simulink model "simulinkmodel"  (R2023a)
settings: Solver=ode4  StartTime=0.0  StopTime=250.0  FixedStep=1e-3  RelTol=1e-3
values from neighbouring files (symbols this model uses):
  ARw = 7.9456    [EOMs_of_AC.m]    (also in constants_simulinkmodel.m)
  b = 9.16    [EOMs_of_AC.m]    (also in constants_simulinkmodel.m)
  c = 1.3333    [EOMs_of_AC.m]    (also in constants_simulinkmodel.m)
  CDf = .005    (= 0.005)    [EOMs_of_AC.m]    (also in constants_simulinkmodel.m)
  CDmint = .002    (= 0.002)    [EOMs_of_AC.m]    (also in constants_simulinkmodel.m)
  CDminvt = .001    (= 0.001)    [EOMs_of_AC.m]    (also in constants_simulinkmodel.m)
  CDminw = .011    (= 0.011)    [EOMs_of_AC.m]    (also in constants_simulinkmodel.m)
  cgt = 3.5    [EOMs_of_AC.m]    (also in constants_simulinkmodel.m)
  cgvt = cgt    (= 3.5)    [EOMs_of_AC.m]    (also in constants_simulinkmodel.m)
  cgw = -.416    (= -0.416)    [EOMs_of_AC.m]    (also in constants_simulinkmodel.m)
  CLat = .76    (= 0.76)    [EOMs_of_AC.m]    (also in constants_simulinkmodel.m)
  CLavt = .0969    (= 0.0969)    [EOMs_of_AC.m]    (also in constants_simulinkmodel.m)
  CLaw = 4.59    [EOMs_of_AC.m]    (also in constants_simulinkmodel.m)
  Clb = -.1    (= -0.1)    [EOMs_of_AC.m]    (also in constants_simulinkmodel.m)
  Clda = 0.244    [EOMs_of_AC.m]    (also in constants_simulinkmodel.m)
  CLow = .421    (= 0.421)    [EOMs_of_AC.m]    (also in constants_simulinkmodel.m)
  Clr = .01    (= 0.01)    [EOMs_of_AC.m]    (also in constants_simulinkmodel.m)
  Cmaf = .114    (= 0.114)    [EOMs_of_AC.m]    (also in constants_simulinkmodel.m)
  Cmw = -0.005    [EOMs_of_AC.m]    (also in constants_simulinkmodel.m)
  Cnda = -0.0128    [EOMs_of_AC.m]    (also in constants_simulinkmodel.m)
  e = .75    (= 0.75)    [EOMs_of_AC.m]    (also in constants_simulinkmodel.m)
  g = 32.17    [EOMs_of_AC.m]    (also in constants_simulinkmodel.m)
  it = 2*d2r    (= 0.0349065850399)    [EOMs_of_AC.m]    (also in constants_simulinkmodel.m = 0.034906585)
  Ixx = 1.9480    (= 1.948)    [EOMs_of_AC.m]    (also in constants_simulinkmodel.m)
  Iyy = 1.5523    [EOMs_of_AC.m]    (also in constants_simulinkmodel.m)
  Izz = 1.9166    [EOMs_of_AC.m]    (also in constants_simulinkmodel.m)
  Kt = .446    (= 0.446)    [EOMs_of_AC.m]    (also in constants_simulinkmodel.m)
  lambda = .72955    (= 0.72955)    [EOMs_of_AC.m]    (also in constants_simulinkmodel.m)
  m = .487669    (= 0.487669)    [EOMs_of_AC.m]    (also in constants_simulinkmodel.m)
  nt = 1    [EOMs_of_AC.m]    (also in constants_simulinkmodel.m)
  nvt = nt    (= 1)    [EOMs_of_AC.m]    (also in constants_simulinkmodel.m)
  rho = .0023081    (= 0.0023081)    [EOMs_of_AC.m]    (also in constants_simulinkmodel.m)
  S = 10.56    [EOMs_of_AC.m]    (also in constants_simulinkmodel.m)
  St = S    (= 10.56)    [EOMs_of_AC.m]    (also in constants_simulinkmodel.m)
  Svt = S    (= 10.56)    [EOMs_of_AC.m]    (also in constants_simulinkmodel.m)
  Te = .422    (= 0.422)    [EOMs_of_AC.m]    (also in constants_simulinkmodel.m)
  Tr = .434    (= 0.434)    [EOMs_of_AC.m]    (also in constants_simulinkmodel.m)
undefined symbols (not defined in the file or in its folder): JSBSim, Rascal110, x_initial
libraries: simulink_extras x12, aerolibfltsims x2, aerolibanimutils x1
(part 2 of 2)

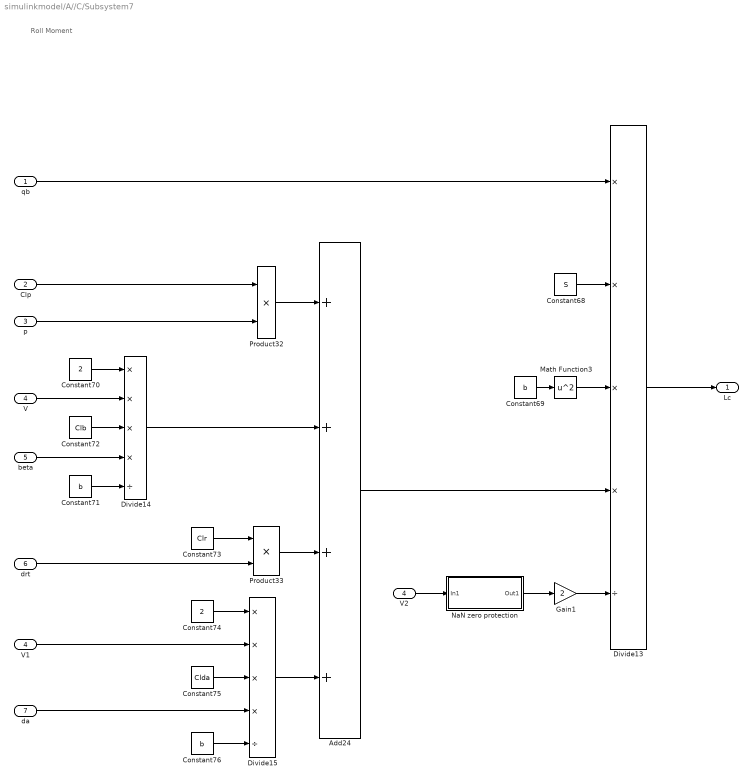
== system simulinkmodel/A//C/Subsystem7 ==
  note: Roll Moment
  qb : Inport
  Clp : Inport  Port=2
  p : Inport  Port=3
  V : Inport  Port=4
  beta : Inport  Port=5
  drt : Inport  Port=6
  da : Inport  Port=7
  Add24 : Sum  Inputs=++++
  Constant68 : Constant  Value=S
  Constant69 : Constant  Value=b
  Constant70 : Constant  Value=2
  Constant71 : Constant  Value=b
  Constant72 : Constant  Value=Clb
  Constant73 : Constant  Value=Clr
  Constant74 : Constant  Value=2
  Constant75 : Constant  Value=Clda
  Constant76 : Constant  Value=b
  Divide13 : Product  Inputs=****/
  Divide14 : Product  Inputs=****/
  Divide15 : Product  Inputs=****/
  Gain1 : Gain  Gain=2
  Math Function3 : Math  Operator=square
  NaN zero protection : Subsystem
  Product32 : Product
  Product33 : Product
  V1 : InportShadow  Port=4
  V2 : InportShadow  Port=4
  Lc : Outport
  wires:
  Add24/1 -> Divide13/4
  Constant72/1 -> Divide14/3
  Math Function3/1 -> Divide13/3
  Constant68/1 -> Divide13/2
  Gain1/1 -> Divide13/5
  Constant73/1 -> Product33/1
  Constant75/1 -> Divide15/3
  Divide14/1 -> Add24/2
  Constant74/1 -> Divide15/1
  Constant69/1 -> Math Function3/1
  Constant76/1 -> Divide15/5
  Product33/1 -> Add24/3
  Divide15/1 -> Add24/4
  qb/1 -> Divide13/1
  Constant71/1 -> Divide14/5
  Product32/1 -> Add24/1
  NaN zero protection/1(Out1) -> Gain1/1
  Constant70/1 -> Divide14/1
  Divide13/1 -> Lc/1
  drt/1 -> Product33/2
  beta/1 -> Divide14/4
  V/1 -> Divide14/2
  da/1 -> Divide15/4
  V1/1 -> Divide15/2
  Clp/1 -> Product32/1
  V2/1 -> NaN zero protection/1(In1)
  p/1 -> Product32/2

== system simulinkmodel/A//C/Subsystem8 ==
  note: Acceleration
  D : Inport
  beta : Inport  Port=2
  Y : Inport  Port=3
  T : Inport  Port=4
  alpha : Inport  Port=5
  gamma : Inport  Port=6
  Add25 : Sum  Inputs=+-
  Add26 : Sum  Inputs=-++
  Constant77 : Constant  Value=g
  Constant78 : Constant  Value=m
  Divide16 : Product  Inputs=*/
  Product34 : Product
  Product35 : Product
  Product36 : Product
  Product37 : Product  Inputs=3
  Trigonometric Function10 : Trigonometry
  Trigonometric Function11 : Trigonometry  Operator=cos
  Trigonometric Function12 : Trigonometry  Operator=cos
  Trigonometric Function8 : Trigonometry
  Trigonometric Function9 : Trigonometry  Operator=cos
  beta1 : InportShadow  Port=2
  beta2 : InportShadow  Port=2
  V_dot : Outport
  wires:
  Trigonometric Function8/1 -> Product34/2
  Constant77/1 -> Product34/1
  Product34/1 -> Add25/2
  Trigonometric Function12/1 -> Product37/3
  Product36/1 -> Add26/2
  Constant78/1 -> Divide16/2
  Divide16/1 -> Add25/1
  Product35/1 -> Add26/1
  Trigonometric Function11/1 -> Product37/2
  Product37/1 -> Add26/3
  Add26/1 -> Divide16/1
  Y/1 -> Product36/1
  Trigonometric Function10/1 -> Product36/2
  Trigonometric Function9/1 -> Product35/2
  Add25/1 -> V_dot/1
  D/1 -> Product35/1
  beta1/1 -> Trigonometric Function10/1
  gamma/1 -> Trigonometric Function8/1
  T/1 -> Product37/1
  beta/1 -> Trigonometric Function9/1
  beta2/1 -> Trigonometric Function11/1
  alpha/1 -> Trigonometric Function12/1

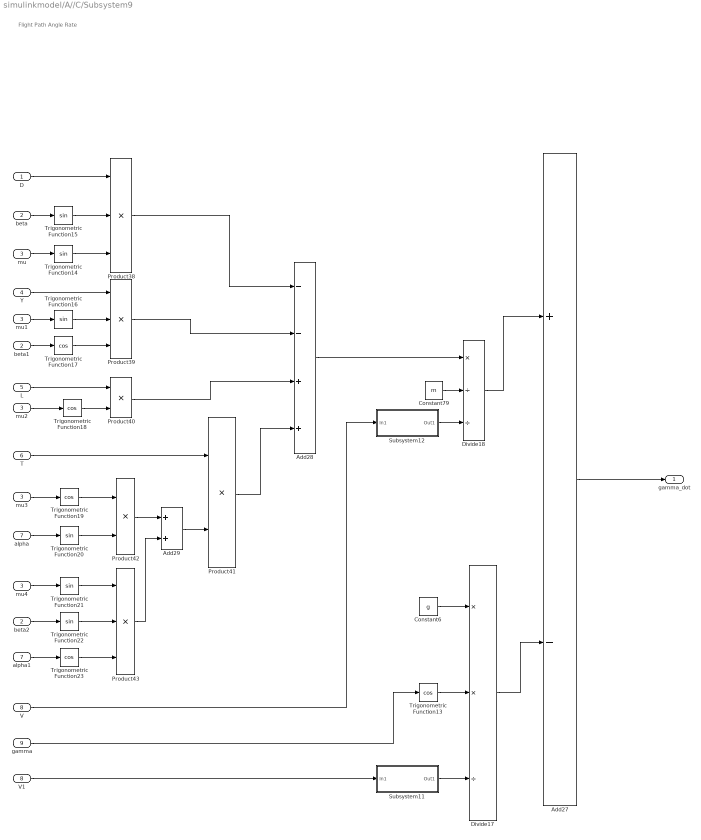
== system simulinkmodel/A//C/Subsystem9 ==
  note: Flight Path Angle Rate
  D : Inport
  beta : Inport  Port=2
  mu : Inport  Port=3
  Y : Inport  Port=4
  L : Inport  Port=5
  T : Inport  Port=6
  alpha : Inport  Port=7
  V : Inport  Port=8
  gamma : Inport  Port=9
  Add27 : Sum  Inputs=+-
  Add28 : Sum  Inputs=--++
  Add29 : Sum
  Constant6 : Constant  Value=g
  Constant79 : Constant  Value=m
  Divide17 : Product  Inputs=**/
  Divide18 : Product  Inputs=*//
  Product38 : Product  Inputs=3
  Product39 : Product  Inputs=3
  Product40 : Product
  Product41 : Product
  Product42 : Product
  Product43 : Product  Inputs=3
  Subsystem11 : Subsystem
  Subsystem12 : Subsystem
  Trigonometric Function{13,17..19,23} (5 alike) : Trigonometry  Operator=cos
  Trigonometric Function{14..16,20..22} (6 alike) : Trigonometry
  V1 : InportShadow  Port=8
  alpha1 : InportShadow  Port=7
  beta1 : InportShadow  Port=2
  beta2 : InportShadow  Port=2
  mu{1..4} (4 alike) : InportShadow  Port=3
  gamma_dot : Outport
  wires:
  alpha/1 -> Trigonometric Function20/1
  Product41/1 -> Add28/4
  Product38/1 -> Add28/1
  Constant6/1 -> Divide17/1
  Divide17/1 -> Add27/2
  mu2/1 -> Trigonometric Function18/1
  Trigonometric Function23/1 -> Product43/3
  Add29/1 -> Product41/2
  Trigonometric Function15/1 -> Product38/2
  Trigonometric Function14/1 -> Product38/3
  Trigonometric Function18/1 -> Product40/2
  Product39/1 -> Add28/2
  mu1/1 -> Trigonometric Function16/1
  Product40/1 -> Add28/3
  Trigonometric Function16/1 -> Product39/2
  V1/1 -> Subsystem11/1(In1)
  alpha1/1 -> Trigonometric Function23/1
  Add28/1 -> Divide18/1
  mu/1 -> Trigonometric Function14/1
  Trigonometric Function17/1 -> Product39/3
  Constant79/1 -> Divide18/2
  Subsystem11/1(Out1) -> Divide17/3
  Trigonometric Function22/1 -> Product43/2
  beta2/1 -> Trigonometric Function22/1
  Product43/1 -> Add29/2
  L/1 -> Product40/1
  Product42/1 -> Add29/1
  Divide18/1 -> Add27/1
  Trigonometric Function20/1 -> Product42/2
  Trigonometric Function13/1 -> Divide17/2
  Trigonometric Function21/1 -> Product43/1
  Trigonometric Function19/1 -> Product42/1
  mu3/1 -> Trigonometric Function19/1
  Subsystem12/1(Out1) -> Divide18/3
  gamma/1 -> Trigonometric Function13/1
  beta/1 -> Trigonometric Function15/1
  D/1 -> Product38/1
  T/1 -> Product41/1
  beta1/1 -> Trigonometric Function17/1
  V/1 -> Subsystem12/1(In1)
  mu4/1 -> Trigonometric Function21/1
  Add27/1 -> gamma_dot/1
  Y/1 -> Product39/1

== system simulinkmodel/Subsystem1/Subsystem ==
  note: Meridian Radius
  latitude : Inport
  Add : Sum  Inputs=+-
  Add1 : Sum  Inputs=+-
  Constant : Constant
  Constant1 : Constant
  Constant2 : Constant  Value=3/2
  Divide : Product  Inputs=**/
  Math Function : Math  Operator=square
  Math Function1 : Math  Operator=square
  Math Function2 : Math  Operator=square
  Math Function3 : Math  Operator=pow
  Product : Product
  Trigonometric Function : Trigonometry
  a (equitorial radius) : Constant  Value=6378137
  e (first eccentricity) : Constant  Value=0.081819190842622
  e (first eccentricity)1 : Constant  Value=0.081819190842622
  M : Outport
  wires:
  Constant1/1 -> Add1/1
  Add/1 -> Divide/2
  Add1/1 -> Math Function3/1
  Constant2/1 -> Math Function3/2
  Product/1 -> Add1/2
  a (equitorial radius)/1 -> Divide/1
  e (first eccentricity)1/1 -> Math Function1/1
  latitude/1 -> Trigonometric Function/1
  Math Function/1 -> Add/2
  Constant/1 -> Add/1
  Trigonometric Function/1 -> Math Function2/1
  e (first eccentricity)/1 -> Math Function/1
  Math Function1/1 -> Product/1
  Math Function2/1 -> Product/2
  Math Function3/1 -> Divide/3
  Divide/1 -> M/1

== system simulinkmodel/Subsystem1/Subsystem1 ==
  note: Prime Vertical Radius
  latitude : Inport
  Add1 : Sum  Inputs=+-
  Constant1 : Constant
  Constant2 : Constant  Value=1/2
  Divide : Product  Inputs=*/
  Math Function1 : Math  Operator=square
  Math Function2 : Math  Operator=square
  Math Function3 : Math  Operator=pow
  Product : Product
  Trigonometric Function : Trigonometry
  a (equitorial radius) : Constant  Value=6378137
  e (first eccentricity) : Constant  Value=0.081819190842622
  N : Outport
  wires:
  Math Function1/1 -> Product/1
  Product/1 -> Add1/2
  Constant2/1 -> Math Function3/2
  Constant1/1 -> Add1/1
  Add1/1 -> Math Function3/1
  latitude/1 -> Trigonometric Function/1
  Math Function3/1 -> Divide/2
  Math Function2/1 -> Product/2
  Trigonometric Function/1 -> Math Function2/1
  e (first eccentricity)/1 -> Math Function1/1
  a (equitorial radius)/1 -> Divide/1
  Divide/1 -> N/1

== system simulinkmodel/Subsystem1/Subsystem2 ==
  note: Latitude Rate
  n_dot : Inport
  M : Inport  Port=2
  h : Inport  Port=3
  Add : Sum
  Divide : Product  Inputs=*/
  ft2m1 : Gain  Gain=0.3048
  latitude_dot : Outport
  wires:
  Add/1 -> Divide/2
  n_dot/1 -> ft2m1/1
  Divide/1 -> latitude_dot/1
  M/1 -> Add/1
  ft2m1/1 -> Divide/1
  h/1 -> Add/2

== system simulinkmodel/Subsystem1/Subsystem3 ==
  note: Longitude Rate
  e_dot : Inport
  N : Inport  Port=2
  h : Inport  Port=3
  latitude : Inport  Port=4
  Add : Sum
  Divide : Product  Inputs=*//
  Gain1 : Gain  Gain=0.3048
  Trigonometric Function : Trigonometry  Operator=cos
  longitude_dot : Outport
  wires:
  Trigonometric Function/1 -> Divide/3
  Divide/1 -> longitude_dot/1
  Add/1 -> Divide/2
  e_dot/1 -> Gain1/1
  latitude/1 -> Trigonometric Function/1
  N/1 -> Add/1
  Gain1/1 -> Divide/1
  h/1 -> Add/2

== system simulinkmodel/Subsystem1/Subsystem4 ==
  note: Altitude Rate
  d_dot : Inport
  Gain : Gain  Gain=-1
  ft2m : Gain  Gain=0.3048
  h_dot : Outport
  wires:
  d_dot/1 -> ft2m/1
  Gain/1 -> h_dot/1
  ft2m/1 -> Gain/1

== system simulinkmodel/A//C/Subsystem10/Subsystem13 ==
  In1 : Inport
  Constant : Constant  Value=1e-8
  Relational Operator : RelationalOperator  Operator=>  OutDataTypeStr=boolean  RndMeth=Simplest  InputSameDT=off
  Switch : Switch  Criteria=u2 ~= 0  SaturateOnIntegerOverflow=off  InputSameDT=off
  Out1 : Outport
  wires:
  Switch/1 -> Out1/1
  Relational Operator/1 -> Switch/2
  Constant/1 -> Relational Operator/2, Switch/3
  In1/1 -> Relational Operator/1, Switch/1

== system simulinkmodel/A//C/Subsystem10/Subsystem14 ==
  In1 : Inport
  Constant : Constant  Value=1e-8
  Relational Operator : RelationalOperator  Operator=>  OutDataTypeStr=boolean  RndMeth=Simplest  InputSameDT=off
  Switch : Switch  Criteria=u2 ~= 0  SaturateOnIntegerOverflow=off  InputSameDT=off
  Out1 : Outport
  wires:
  In1/1 -> Switch/1, Relational Operator/1
  Constant/1 -> Switch/3, Relational Operator/2
  Relational Operator/1 -> Switch/2
  Switch/1 -> Out1/1

== system simulinkmodel/A//C/Subsystem14/Subsystem15 ==
  In1 : Inport
  Constant : Constant  Value=1e-8
  Relational Operator : RelationalOperator  Operator=>  OutDataTypeStr=boolean  RndMeth=Simplest  InputSameDT=off
  Switch : Switch  Criteria=u2 ~= 0  SaturateOnIntegerOverflow=off  InputSameDT=off
  Out1 : Outport
  wires:
  Switch/1 -> Out1/1
  Relational Operator/1 -> Switch/2
  Constant/1 -> Relational Operator/2, Switch/3
  In1/1 -> Relational Operator/1, Switch/1

== system simulinkmodel/A//C/Subsystem14/Subsystem16 ==
  In1 : Inport
  Constant : Constant  Value=1e-8
  Relational Operator : RelationalOperator  Operator=>  OutDataTypeStr=boolean  RndMeth=Simplest  InputSameDT=off
  Switch : Switch  Criteria=u2 ~= 0  SaturateOnIntegerOverflow=off  InputSameDT=off
  Out1 : Outport
  wires:
  In1/1 -> Switch/1, Relational Operator/1
  Constant/1 -> Switch/3, Relational Operator/2
  Relational Operator/1 -> Switch/2
  Switch/1 -> Out1/1

== system simulinkmodel/A//C/Subsystem15/Subsystem17 ==
  In1 : Inport
  Constant : Constant  Value=1e-8
  Relational Operator : RelationalOperator  Operator=>  OutDataTypeStr=boolean  RndMeth=Simplest  InputSameDT=off
  Switch : Switch  Criteria=u2 ~= 0  SaturateOnIntegerOverflow=off  InputSameDT=off
  Out1 : Outport
  wires:
  In1/1 -> Switch/1, Relational Operator/1
  Constant/1 -> Switch/3, Relational Operator/2
  Relational Operator/1 -> Switch/2
  Switch/1 -> Out1/1

== system simulinkmodel/A//C/Subsystem15/Subsystem18 ==
  V : Inport
  Constant : Constant  Value=1e-8
  Relational Operator : RelationalOperator  Operator=>  OutDataTypeStr=boolean  RndMeth=Simplest  InputSameDT=off
  Switch : Switch  Criteria=u2 ~= 0  SaturateOnIntegerOverflow=off  InputSameDT=off
  Out1 : Outport
  wires:
  Switch/1 -> Out1/1
  Relational Operator/1 -> Switch/2
  Constant/1 -> Relational Operator/2, Switch/3
  V/1 -> Relational Operator/1, Switch/1

== system simulinkmodel/A//C/Subsystem2/Subsystem1 ==
  In1 : Inport
  Constant : Constant  Value=1e-8
  Relational Operator : RelationalOperator  Operator=>  OutDataTypeStr=boolean  RndMeth=Simplest  InputSameDT=off
  Switch : Switch  Criteria=u2 ~= 0  SaturateOnIntegerOverflow=off  InputSameDT=off
  Out1 : Outport
  wires:
  Switch/1 -> Out1/1
  Relational Operator/1 -> Switch/2
  Constant/1 -> Relational Operator/2, Switch/3
  In1/1 -> Relational Operator/1, Switch/1

== system simulinkmodel/A//C/Subsystem25/Subsystem2 ==
  In1 : Inport
  Constant : Constant  Value=1e-8
  Relational Operator : RelationalOperator  Operator=>  OutDataTypeStr=boolean  RndMeth=Simplest  InputSameDT=off
  Switch : Switch  Criteria=u2 ~= 0  SaturateOnIntegerOverflow=off  InputSameDT=off
  Out1 : Outport
  wires:
  In1/1 -> Switch/1, Relational Operator/1
  Constant/1 -> Switch/3, Relational Operator/2
  Relational Operator/1 -> Switch/2
  Switch/1 -> Out1/1

== system simulinkmodel/A//C/Subsystem3/Subsystem5 ==
  In1 : Inport
  Constant : Constant  Value=1e-8
  Relational Operator : RelationalOperator  Operator=>  OutDataTypeStr=boolean  RndMeth=Simplest  InputSameDT=off
  Switch : Switch  Criteria=u2 ~= 0  SaturateOnIntegerOverflow=off  InputSameDT=off
  Out1 : Outport
  wires:
  In1/1 -> Switch/1, Relational Operator/1
  Constant/1 -> Switch/3, Relational Operator/2
  Relational Operator/1 -> Switch/2
  Switch/1 -> Out1/1

== system simulinkmodel/A//C/Subsystem3/Subsystem6 ==
  In1 : Inport
  Constant : Constant  Value=1e-8
  Relational Operator : RelationalOperator  Operator=>  OutDataTypeStr=boolean  RndMeth=Simplest  InputSameDT=off
  Switch : Switch  Criteria=u2 ~= 0  SaturateOnIntegerOverflow=off  InputSameDT=off
  Out1 : Outport
  wires:
  Switch/1 -> Out1/1
  Relational Operator/1 -> Switch/2
  Constant/1 -> Relational Operator/2, Switch/3
  In1/1 -> Relational Operator/1, Switch/1

== system simulinkmodel/A//C/Subsystem35/Subsystem3 ==
  In1 : Inport
  Constant : Constant  Value=1e-8
  Relational Operator : RelationalOperator  Operator=>  OutDataTypeStr=boolean  RndMeth=Simplest  InputSameDT=off
  Switch : Switch  Criteria=u2 ~= 0  SaturateOnIntegerOverflow=off  InputSameDT=off
  Out1 : Outport
  wires:
  Switch/1 -> Out1/1
  Relational Operator/1 -> Switch/2
  Constant/1 -> Relational Operator/2, Switch/3
  In1/1 -> Relational Operator/1, Switch/1

== system simulinkmodel/A//C/Subsystem35/Subsystem4 ==
  In1 : Inport
  Constant : Constant  Value=1e-8
  Relational Operator : RelationalOperator  Operator=>  OutDataTypeStr=boolean  RndMeth=Simplest  InputSameDT=off
  Switch : Switch  Criteria=u2 ~= 0  SaturateOnIntegerOverflow=off  InputSameDT=off
  Out1 : Outport
  wires:
  In1/1 -> Switch/1, Relational Operator/1
  Constant/1 -> Switch/3, Relational Operator/2
  Relational Operator/1 -> Switch/2
  Switch/1 -> Out1/1

== system simulinkmodel/A//C/Subsystem36/Subsystem19 ==
  In1 : Inport
  Constant : Constant  Value=1e-8
  Relational Operator : RelationalOperator  Operator=>  OutDataTypeStr=boolean  RndMeth=Simplest  InputSameDT=off
  Switch : Switch  Criteria=u2 ~= 0  SaturateOnIntegerOverflow=off  InputSameDT=off
  Out1 : Outport
  wires:
  Switch/1 -> Out1/1
  Relational Operator/1 -> Switch/2
  Constant/1 -> Relational Operator/2, Switch/3
  In1/1 -> Relational Operator/1, Switch/1

== system simulinkmodel/A//C/Subsystem4/Subsystem7 ==
  In1 : Inport
  Constant : Constant  Value=1e-8
  Relational Operator : RelationalOperator  Operator=>  OutDataTypeStr=boolean  RndMeth=Simplest  InputSameDT=off
  Switch : Switch  Criteria=u2 ~= 0  SaturateOnIntegerOverflow=off  InputSameDT=off
  Out1 : Outport
  wires:
  In1/1 -> Switch/1, Relational Operator/1
  Constant/1 -> Switch/3, Relational Operator/2
  Relational Operator/1 -> Switch/2
  Switch/1 -> Out1/1

== system simulinkmodel/A//C/Subsystem5/Subsystem8 ==
  In1 : Inport
  Constant : Constant  Value=1e-8
  Relational Operator : RelationalOperator  Operator=>  OutDataTypeStr=boolean  RndMeth=Simplest  InputSameDT=off
  Switch : Switch  Criteria=u2 ~= 0  SaturateOnIntegerOverflow=off  InputSameDT=off
  Out1 : Outport
  wires:
  In1/1 -> Switch/1, Relational Operator/1
  Constant/1 -> Switch/3, Relational Operator/2
  Relational Operator/1 -> Switch/2
  Switch/1 -> Out1/1

== system simulinkmodel/A//C/Subsystem5/Subsystem9 ==
  In1 : Inport
  Constant : Constant  Value=1e-8
  Relational Operator : RelationalOperator  Operator=>  OutDataTypeStr=boolean  RndMeth=Simplest  InputSameDT=off
  Switch : Switch  Criteria=u2 ~= 0  SaturateOnIntegerOverflow=off  InputSameDT=off
  Out1 : Outport
  wires:
  Switch/1 -> Out1/1
  Relational Operator/1 -> Switch/2
  Constant/1 -> Relational Operator/2, Switch/3
  In1/1 -> Relational Operator/1, Switch/1

== system simulinkmodel/A//C/Subsystem6/Subsystem10 ==
  In1 : Inport
  Constant : Constant  Value=1e-8
  Relational Operator : RelationalOperator  Operator=>  OutDataTypeStr=boolean  RndMeth=Simplest  InputSameDT=off
  Switch : Switch  Criteria=u2 ~= 0  SaturateOnIntegerOverflow=off  InputSameDT=off
  Out1 : Outport
  wires:
  In1/1 -> Switch/1, Relational Operator/1
  Constant/1 -> Switch/3, Relational Operator/2
  Relational Operator/1 -> Switch/2
  Switch/1 -> Out1/1

== system simulinkmodel/A//C/Subsystem7/NaN zero protection ==
  In1 : Inport
  Constant : Constant  Value=1e-8
  Relational Operator : RelationalOperator  Operator=>  OutDataTypeStr=boolean  RndMeth=Simplest  InputSameDT=off
  Switch : Switch  Criteria=u2 ~= 0  SaturateOnIntegerOverflow=off  InputSameDT=off
  Out1 : Outport
  wires:
  Switch/1 -> Out1/1
  Relational Operator/1 -> Switch/2
  Constant/1 -> Relational Operator/2, Switch/3
  In1/1 -> Relational Operator/1, Switch/1

== system simulinkmodel/A//C/Subsystem9/Subsystem11 ==
  In1 : Inport
  Constant : Constant  Value=1e-8
  Relational Operator : RelationalOperator  Operator=>  OutDataTypeStr=boolean  RndMeth=Simplest  InputSameDT=off
  Switch : Switch  Criteria=u2 ~= 0  SaturateOnIntegerOverflow=off  InputSameDT=off
  Out1 : Outport
  wires:
  In1/1 -> Switch/1, Relational Operator/1
  Constant/1 -> Switch/3, Relational Operator/2
  Relational Operator/1 -> Switch/2
  Switch/1 -> Out1/1

== system simulinkmodel/A//C/Subsystem9/Subsystem12 ==
  In1 : Inport
  Constant : Constant  Value=1e-8
  Relational Operator : RelationalOperator  Operator=>  OutDataTypeStr=boolean  RndMeth=Simplest  InputSameDT=off
  Switch : Switch  Criteria=u2 ~= 0  SaturateOnIntegerOverflow=off  InputSameDT=off
  Out1 : Outport
  wires:
  Switch/1 -> Out1/1
  Relational Operator/1 -> Switch/2
  Constant/1 -> Relational Operator/2, Switch/3
  In1/1 -> Relational Operator/1, Switch/1
